simulink model "PHASE6_ASHUGANJ_CCPP_CLOSED_LOOP_TRIP"  (R2024a)
settings: Solver=FixedStepDiscrete  StartTime=0  StopTime=2  FixedStep=5e-05  RelTol=1e-3
PostLoadFcn:
  | p6startupdir=fileparts(get_param(bdroot,'FileName')); while ~isfile(fullfile(p6startupdir,'scripts','setup_phase6_workspace.m')), p6startupparent=fileparts(p6startupdir); assert(~strcmp(p6startupparent,p6startupdir),'Phase6:MissingScripts','Cannot locate the Phase6 scripts folder.'); p6startupdir=p6startupparent; end; addpath(fullfile(p6startupdir,'scripts')); setup_phase6_workspace; clear p6startupdir p6startupparent;
  | phase6_color_wires(bdroot);
StartFcn:
  | phase6_color_wires(bdroot);
StopFcn:
  | phase6_color_wires(bdroot);
model workspace (MAT data in the model file):
  C : object (value not decoded)
  D : object (value not decoded)
  P : object (value not decoded)
  Phase6BuildInfo : object (value not decoded)
  Phase6LoadFlow : object (value not decoded)
  Phase6Metadata : object (value not decoded)
  R : object (value not decoded)
  S : object (value not decoded)
symbols that are objects in the model workspace (value not decoded): C, D, R, S
undefined symbols (not defined in the file): D1, Delta
libraries: spsThreePhaseVIMeasurementLib x18, spsThreePhaseFaultLib x7, spsThreePhaseBreakerLib x5, spsThreePhaseParallelRLCLoadLib x4, spsThreePhasePISectionLineLib x4, spsThreePhaseTransformerTwoWindingsLib x3, spsGroundLib x3, spsSeriesRLCBranchLib x3, spsGroundingTransformerLib x1, spsCurrentMeasurementLib x1, spsSynchronousMachinepuStandardLib x1, spsThreePhaseMutualInductanceZ1Z0Lib x1
(part 2 of 2)

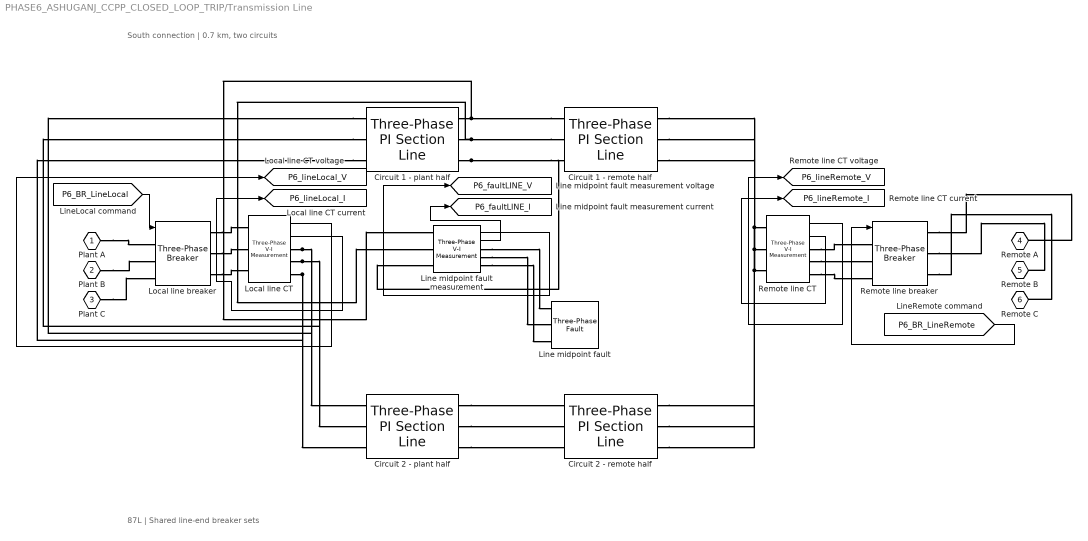
== system PHASE6_ASHUGANJ_CCPP_CLOSED_LOOP_TRIP/Transmission Line ==
  note: South connection | 0.7 km, two circuits
  note: 87L | Shared line-end breaker sets
  Circuit 1 - plant half : spsThreePhasePISectionLineLib/Three-Phase PI Section Line  LConnTagsString=a|b|c  RConnTagsString=A|B|C  Length=0.35  Frequency=50  Resistances=[0.08 0.25]  Inductances=[0.00111408460164327 0.00381971863420549]  Capacitances=[1.33690152197192e-08 8.91267681314614e-09]
  Circuit 1 - remote half : spsThreePhasePISectionLineLib/Three-Phase PI Section Line  LConnTagsString=a|b|c  RConnTagsString=A|B|C  Length=0.35  Frequency=50  Resistances=[0.08 0.25]  Inductances=[0.00111408460164327 0.00381971863420549]  Capacitances=[1.33690152197192e-08 8.91267681314614e-09]
  Circuit 2 - plant half : spsThreePhasePISectionLineLib/Three-Phase PI Section Line  LConnTagsString=a|b|c  RConnTagsString=A|B|C  Length=0.35  Frequency=50  Resistances=[0.08 0.25]  Inductances=[0.00111408460164327 0.00381971863420549]  Capacitances=[1.33690152197192e-08 8.91267681314614e-09]
  Circuit 2 - remote half : spsThreePhasePISectionLineLib/Three-Phase PI Section Line  LConnTagsString=a|b|c  RConnTagsString=A|B|C  Length=0.35  Frequency=50  Resistances=[0.08 0.25]  Inductances=[0.00111408460164327 0.00381971863420549]  Capacitances=[1.33690152197192e-08 8.91267681314614e-09]
  Line midpoint fault : spsThreePhaseFaultLib/Three-Phase Fault  InitialStates=0  FaultA=on  FaultB=on  FaultC=on  GroundFault=off  SwitchTimes=[1000000 1000001]  External=off  SwitchStatus=NaN  FaultResistance=0.01  GroundResistance=0.01  SnubberResistance=1000000000  SnubberCapacitance=inf  Measurements=None
  Line midpoint fault measurement : spsThreePhaseVIMeasurementLib/Three-Phase V-I Measurement  VoltageMeasurement=phase-to-ground  SetLabelV=off  LabelV=Vabc  Vpu=off  VpuLL=off  CurrentMeasurement=yes  SetLabelI=off  LabelI=Iabc  Ipu=off  Pbase=100e6  Vbase=500e3  OutputType=Complex  PhasorSimulation=off  PSBequivalent=0
  Local line CT : spsThreePhaseVIMeasurementLib/Three-Phase V-I Measurement  VoltageMeasurement=phase-to-ground  SetLabelV=off  LabelV=Vabc  Vpu=off  VpuLL=off  CurrentMeasurement=yes  SetLabelI=off  LabelI=Iabc  Ipu=off  Pbase=100e6  Vbase=500e3  OutputType=Complex  PhasorSimulation=off  PSBequivalent=0
  Local line breaker : spsThreePhaseBreakerLib/Three-Phase Breaker  InitialState=closed  SwitchA=on  SwitchB=on  SwitchC=on  SwitchTimes="[1/60  5/60]"  External=on  BreakerResistance=0.0001  SnubberResistance=1000000  SnubberCapacitance=inf  Measurements=None
  Remote line CT : spsThreePhaseVIMeasurementLib/Three-Phase V-I Measurement  VoltageMeasurement=phase-to-ground  SetLabelV=off  LabelV=Vabc  Vpu=off  VpuLL=off  CurrentMeasurement=yes  SetLabelI=off  LabelI=Iabc  Ipu=off  Pbase=100e6  Vbase=500e3  OutputType=Complex  PhasorSimulation=off  PSBequivalent=0
  Remote line breaker : spsThreePhaseBreakerLib/Three-Phase Breaker  InitialState=closed  SwitchA=on  SwitchB=on  SwitchC=on  SwitchTimes="[1/60  5/60]"  External=on  BreakerResistance=0.0001  SnubberResistance=1000000  SnubberCapacitance=inf  Measurements=None
  Plant A : PMIOPort  Side=Left
  Plant B : PMIOPort  Port=2  Side=Left
  Plant C : PMIOPort  Port=3  Side=Left
  Remote A : PMIOPort  Port=4  Side=Right
  Remote B : PMIOPort  Port=5  Side=Right
  Remote C : PMIOPort  Port=6  Side=Right
  tag scope: P6_faultLINE_I=global, P6_faultLINE_V=global, P6_lineLocal_I=global, P6_lineLocal_V=global, P6_lineRemote_I=global, P6_lineRemote_V=global
  wires:
  [P6_BR_LineLocal] -> Local line breaker/1
  Local line CT/1 -> [P6_lineLocal_V]
  Local line CT/2 -> [P6_lineLocal_I]
  Remote line CT/1 -> [P6_lineRemote_V]
  Remote line CT/2 -> [P6_lineRemote_I]
  [P6_BR_LineRemote] -> Remote line breaker/1
  Line midpoint fault measurement/1 -> [P6_faultLINE_V]
  Line midpoint fault measurement/2 -> [P6_faultLINE_I]
  connections:
  Plant A/RConn1 -- Local line breaker/LConn1
  Plant B/RConn1 -- Local line breaker/LConn2
  Plant C/RConn1 -- Local line breaker/LConn3
  Local line breaker/RConn1 -- Local line CT/LConn1
  Local line breaker/RConn2 -- Local line CT/LConn2
  Local line breaker/RConn3 -- Local line CT/LConn3
  Remote line CT/RConn1 -- Remote line breaker/LConn1
  Remote line CT/RConn2 -- Remote line breaker/LConn2
  Remote line CT/RConn3 -- Remote line breaker/LConn3
  Remote line breaker/RConn1 -- Remote A/RConn1
  Remote line breaker/RConn2 -- Remote B/RConn1
  Remote line breaker/RConn3 -- Remote C/RConn1
  Circuit 1 - plant half/LConn1 -- Local line CT/RConn1 -- Circuit 2 - plant half/LConn1
  Circuit 1 - plant half/LConn2 -- Local line CT/RConn2 -- Circuit 2 - plant half/LConn2
  Circuit 1 - plant half/LConn3 -- Local line CT/RConn3 -- Circuit 2 - plant half/LConn3
  Circuit 1 - remote half/LConn1 -- Circuit 1 - plant half/RConn1 -- Line midpoint fault measurement/LConn1
  Circuit 1 - remote half/LConn2 -- Circuit 1 - plant half/RConn2 -- Line midpoint fault measurement/LConn2
  Circuit 1 - remote half/LConn3 -- Circuit 1 - plant half/RConn3 -- Line midpoint fault measurement/LConn3
  Remote line CT/LConn1 -- Circuit 1 - remote half/RConn1 -- Circuit 2 - remote half/RConn1
  Remote line CT/LConn2 -- Circuit 1 - remote half/RConn2 -- Circuit 2 - remote half/RConn2
  Remote line CT/LConn3 -- Circuit 1 - remote half/RConn3 -- Circuit 2 - remote half/RConn3
  Line midpoint fault measurement/RConn1 -- Line midpoint fault/LConn1
  Line midpoint fault measurement/RConn2 -- Line midpoint fault/LConn2
  Line midpoint fault measurement/RConn3 -- Line midpoint fault/LConn3
  Circuit 2 - plant half/RConn1 -- Circuit 2 - remote half/LConn1
  Circuit 2 - plant half/RConn2 -- Circuit 2 - remote half/LConn2
  Circuit 2 - plant half/RConn3 -- Circuit 2 - remote half/LConn3

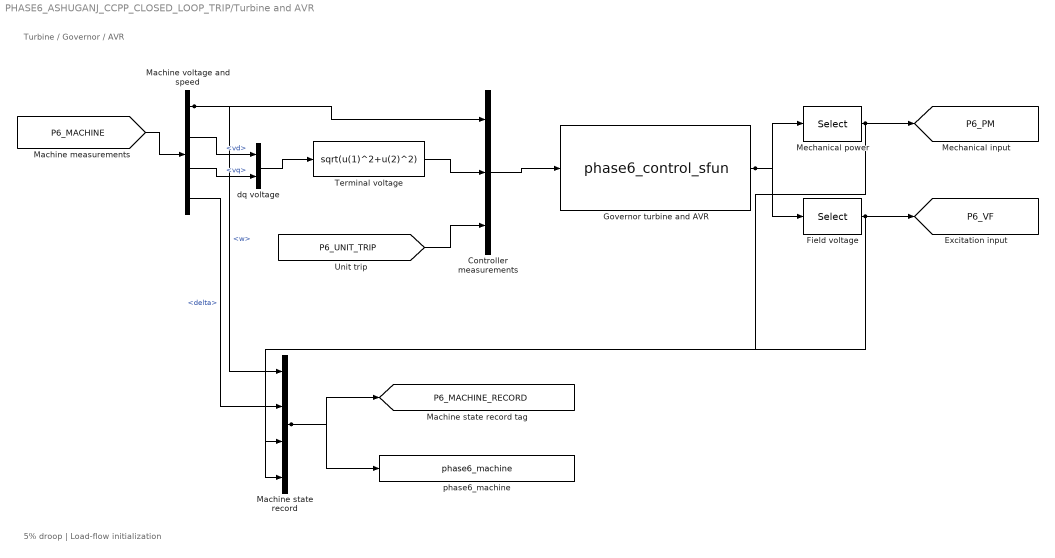
== system PHASE6_ASHUGANJ_CCPP_CLOSED_LOOP_TRIP/Turbine and AVR ==
  note: Turbine / Governor / AVR
  note: 5% droop | Load-flow initialization
  Controller measurements : Mux  Inputs=3
  Field voltage : Selector  IndexOptions=Index vector (dialog)  Indices=2  OutputSizes=1
  Governor turbine and AVR : M-S-Function  FunctionName=phase6_control_sfun  Parameters=C
  Machine state record : Mux
  Machine voltage and speed : BusSelector  OutputSignals=w,vd,vq,delta
  Mechanical power : Selector  IndexOptions=Index vector (dialog)  Indices=1  OutputSizes=1
  Terminal voltage : Fcn  Expr=sqrt(u(1)^2+u(2)^2)
  dq voltage : Mux  Inputs=2
  phase6_machine : ToWorkspace  VariableName=phase6_machine  SaveFormat=Timeseries  SampleTime=-1
  tag scope: P6_MACHINE_RECORD=global, P6_PM=global, P6_VF=global
  wires:
  [P6_MACHINE] -> Machine voltage and speed/1
  Machine voltage and speed/2 -> dq voltage/1  "<vd>"
  Machine voltage and speed/3 -> dq voltage/2  "<vq>"
  dq voltage/1 -> Terminal voltage/1
  Machine voltage and speed/1 -> Controller measurements/1, Machine state record/1  "<w>"
  Terminal voltage/1 -> Controller measurements/2
  [P6_UNIT_TRIP] -> Controller measurements/3
  Controller measurements/1 -> Governor turbine and AVR/1
  Governor turbine and AVR/1 -> Mechanical power/1, Field voltage/1
  Mechanical power/1 -> [P6_PM], Machine state record/3
  Field voltage/1 -> [P6_VF], Machine state record/4
  Machine voltage and speed/4 -> Machine state record/2  "<delta>"
  Machine state record/1 -> [P6_MACHINE_RECORD], phase6_machine/1

== system PHASE6_ASHUGANJ_CCPP_CLOSED_LOOP_TRIP/Auxiliaries/B6.6 Auxiliary 6.6 kV bus ==
  A1 : PMIOPort  Side=Left
  B1 : PMIOPort  Port=2  Side=Left
  C1 : PMIOPort  Port=3  Side=Left
  A2 : PMIOPort  Port=4  Side=Right
  B2 : PMIOPort  Port=5  Side=Right
  C2 : PMIOPort  Port=6  Side=Right
  connections:
  A1/RConn1 -- A2/RConn1
  B1/RConn1 -- B2/RConn1
  C1/RConn1 -- C2/RConn1

== system PHASE6_ASHUGANJ_CCPP_CLOSED_LOOP_TRIP/Grid/BGRID_230 PGCB 230 kV bus ==
  A1 : PMIOPort  Side=Left
  B1 : PMIOPort  Port=2  Side=Left
  C1 : PMIOPort  Port=3  Side=Left
  A2 : PMIOPort  Port=4  Side=Right
  B2 : PMIOPort  Port=5  Side=Right
  C2 : PMIOPort  Port=6  Side=Right
  connections:
  A1/RConn1 -- A2/RConn1
  B1/RConn1 -- B2/RConn1
  C1/RConn1 -- C2/RConn1

== system PHASE6_ASHUGANJ_CCPP_CLOSED_LOOP_TRIP/Measurements/Auxiliary and neutral ==
  Voltage and current channels : Mux  Inputs=6
  Measured abc : Outport
  wires:
  [P6_aux_V] -> Voltage and current channels/1
  [P6_aux_I] -> Voltage and current channels/2
  [P6_grid_V] -> Voltage and current channels/3
  [P6_grid_I] -> Voltage and current channels/4
  [P6_neutral_V] -> Voltage and current channels/5
  [P6_neutral_I] -> Voltage and current channels/6
  Voltage and current channels/1 -> Measured abc/1

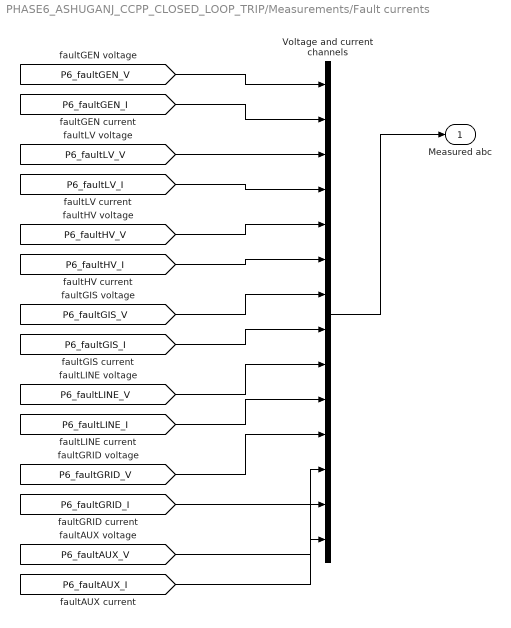
== system PHASE6_ASHUGANJ_CCPP_CLOSED_LOOP_TRIP/Measurements/Fault currents ==
  Voltage and current channels : Mux  Inputs=14
  Measured abc : Outport
  wires:
  [P6_faultGEN_V] -> Voltage and current channels/1
  [P6_faultGEN_I] -> Voltage and current channels/2
  [P6_faultLV_V] -> Voltage and current channels/3
  [P6_faultLV_I] -> Voltage and current channels/4
  [P6_faultHV_V] -> Voltage and current channels/5
  [P6_faultHV_I] -> Voltage and current channels/6
  [P6_faultGIS_V] -> Voltage and current channels/7
  [P6_faultGIS_I] -> Voltage and current channels/8
  [P6_faultLINE_V] -> Voltage and current channels/9
  [P6_faultLINE_I] -> Voltage and current channels/10
  [P6_faultGRID_V] -> Voltage and current channels/11
  [P6_faultGRID_I] -> Voltage and current channels/12
  [P6_faultAUX_V] -> Voltage and current channels/13
  [P6_faultAUX_I] -> Voltage and current channels/14
  Voltage and current channels/1 -> Measured abc/1

== system PHASE6_ASHUGANJ_CCPP_CLOSED_LOOP_TRIP/Measurements/Generator and transformer ==
  Voltage and current channels : Mux  Inputs=8
  Measured abc : Outport
  wires:
  [P6_genInner_V] -> Voltage and current channels/1
  [P6_genInner_I] -> Voltage and current channels/2
  [P6_genTerminal_V] -> Voltage and current channels/3
  [P6_genTerminal_I] -> Voltage and current channels/4
  [P6_gsutLV_V] -> Voltage and current channels/5
  [P6_gsutLV_I] -> Voltage and current channels/6
  [P6_gsutHV_V] -> Voltage and current channels/7
  [P6_gsutHV_I] -> Voltage and current channels/8
  Voltage and current channels/1 -> Measured abc/1

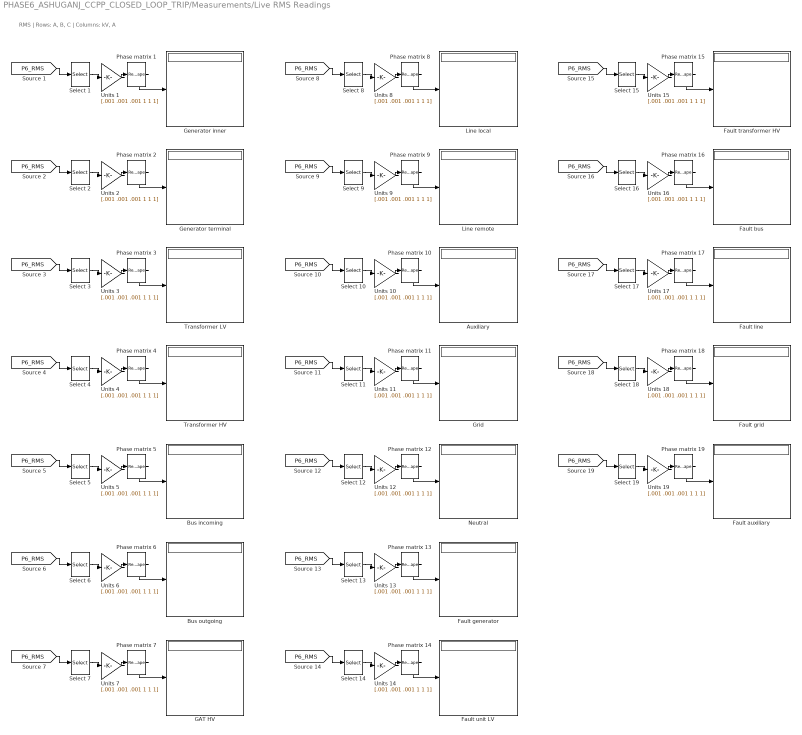
== system PHASE6_ASHUGANJ_CCPP_CLOSED_LOOP_TRIP/Measurements/Live RMS Readings ==
  note: RMS | Rows: A, B, C | Columns: kV, A
  Auxiliary : Display
  Bus incoming : Display
  Bus outgoing : Display
  Fault auxiliary : Display
  Fault bus : Display
  Fault generator : Display
  Fault grid : Display
  Fault line : Display
  Fault transformer HV : Display
  Fault unit LV : Display
  GAT HV : Display
  Generator inner : Display
  Generator terminal : Display
  Grid : Display
  Line local : Display
  Line remote : Display
  Neutral : Display
  Phase matrix {1..19} (19 alike) : Reshape  OutputDimensionality=Customize  OutputDimensions=[3 2]
  Select 1 : Selector  InputPortWidth=114  IndexOptions=Index vector (dialog)  Indices=[1 2 3 4 5 6]  OutputSizes=1
  Select 10 : Selector  InputPortWidth=114  IndexOptions=Index vector (dialog)  Indices=[55 56 57 58 59 60]  OutputSizes=1
  Select 11 : Selector  InputPortWidth=114  IndexOptions=Index vector (dialog)  Indices=[61 62 63 64 65 66]  OutputSizes=1
  Select 12 : Selector  InputPortWidth=114  IndexOptions=Index vector (dialog)  Indices=[67 68 69 70 71 72]  OutputSizes=1
  Select 13 : Selector  InputPortWidth=114  IndexOptions=Index vector (dialog)  Indices=[73 74 75 76 77 78]  OutputSizes=1
  Select 14 : Selector  InputPortWidth=114  IndexOptions=Index vector (dialog)  Indices=[79 80 81 82 83 84]  OutputSizes=1
  Select 15 : Selector  InputPortWidth=114  IndexOptions=Index vector (dialog)  Indices=[85 86 87 88 89 90]  OutputSizes=1
  Select 16 : Selector  InputPortWidth=114  IndexOptions=Index vector (dialog)  Indices=[91 92 93 94 95 96]  OutputSizes=1
  Select 17 : Selector  InputPortWidth=114  IndexOptions=Index vector (dialog)  Indices=[97 98 99 100 101 102]  OutputSizes=1
  Select 18 : Selector  InputPortWidth=114  IndexOptions=Index vector (dialog)  Indices=[103 104 105 106 107 108]  OutputSizes=1
  Select 19 : Selector  InputPortWidth=114  IndexOptions=Index vector (dialog)  Indices=[109 110 111 112 113 114]  OutputSizes=1
  Select 2 : Selector  InputPortWidth=114  IndexOptions=Index vector (dialog)  Indices=[7 8 9 10 11 12]  OutputSizes=1
  Select 3 : Selector  InputPortWidth=114  IndexOptions=Index vector (dialog)  Indices=[13 14 15 16 17 18]  OutputSizes=1
  Select 4 : Selector  InputPortWidth=114  IndexOptions=Index vector (dialog)  Indices=[19 20 21 22 23 24]  OutputSizes=1
  Select 5 : Selector  InputPortWidth=114  IndexOptions=Index vector (dialog)  Indices=[25 26 27 28 29 30]  OutputSizes=1
  Select 6 : Selector  InputPortWidth=114  IndexOptions=Index vector (dialog)  Indices=[31 32 33 34 35 36]  OutputSizes=1
  Select 7 : Selector  InputPortWidth=114  IndexOptions=Index vector (dialog)  Indices=[37 38 39 40 41 42]  OutputSizes=1
  Select 8 : Selector  InputPortWidth=114  IndexOptions=Index vector (dialog)  Indices=[43 44 45 46 47 48]  OutputSizes=1
  Select 9 : Selector  InputPortWidth=114  IndexOptions=Index vector (dialog)  Indices=[49 50 51 52 53 54]  OutputSizes=1
  Transformer HV : Display
  Transformer LV : Display
  Units {1..19} (19 alike) : Gain  Gain=[.001 .001 .001 1 1 1]
  wires:
  [P6_RMS] -> Select 1/1
  Select 1/1 -> Units 1/1
  [P6_RMS] -> Select 2/1
  Select 2/1 -> Units 2/1
  [P6_RMS] -> Select 3/1
  Select 3/1 -> Units 3/1
  [P6_RMS] -> Select 4/1
  Select 4/1 -> Units 4/1
  [P6_RMS] -> Select 5/1
  Select 5/1 -> Units 5/1
  [P6_RMS] -> Select 6/1
  Select 6/1 -> Units 6/1
  [P6_RMS] -> Select 7/1
  Select 7/1 -> Units 7/1
  [P6_RMS] -> Select 8/1
  Select 8/1 -> Units 8/1
  [P6_RMS] -> Select 9/1
  Select 9/1 -> Units 9/1
  [P6_RMS] -> Select 10/1
  Select 10/1 -> Units 10/1
  [P6_RMS] -> Select 11/1
  Select 11/1 -> Units 11/1
  [P6_RMS] -> Select 12/1
  Select 12/1 -> Units 12/1
  [P6_RMS] -> Select 13/1
  Select 13/1 -> Units 13/1
  [P6_RMS] -> Select 14/1
  Select 14/1 -> Units 14/1
  [P6_RMS] -> Select 15/1
  Select 15/1 -> Units 15/1
  [P6_RMS] -> Select 16/1
  Select 16/1 -> Units 16/1
  [P6_RMS] -> Select 17/1
  Select 17/1 -> Units 17/1
  [P6_RMS] -> Select 18/1
  Select 18/1 -> Units 18/1
  [P6_RMS] -> Select 19/1
  Select 19/1 -> Units 19/1
  Units 1/1 -> Phase matrix 1/1
  Phase matrix 1/1 -> Generator inner/1
  Units 2/1 -> Phase matrix 2/1
  Phase matrix 2/1 -> Generator terminal/1
  Units 3/1 -> Phase matrix 3/1
  Phase matrix 3/1 -> Transformer LV/1
  Units 4/1 -> Phase matrix 4/1
  Phase matrix 4/1 -> Transformer HV/1
  Units 5/1 -> Phase matrix 5/1
  Phase matrix 5/1 -> Bus incoming/1
  Units 6/1 -> Phase matrix 6/1
  Phase matrix 6/1 -> Bus outgoing/1
  Units 7/1 -> Phase matrix 7/1
  Phase matrix 7/1 -> GAT HV/1
  Units 8/1 -> Phase matrix 8/1
  Phase matrix 8/1 -> Line local/1
  Units 9/1 -> Phase matrix 9/1
  Phase matrix 9/1 -> Line remote/1
  Units 10/1 -> Phase matrix 10/1
  Phase matrix 10/1 -> Auxiliary/1
  Units 11/1 -> Phase matrix 11/1
  Phase matrix 11/1 -> Grid/1
  Units 12/1 -> Phase matrix 12/1
  Phase matrix 12/1 -> Neutral/1
  Units 13/1 -> Phase matrix 13/1
  Phase matrix 13/1 -> Fault generator/1
  Units 14/1 -> Phase matrix 14/1
  Phase matrix 14/1 -> Fault unit LV/1
  Units 15/1 -> Phase matrix 15/1
  Phase matrix 15/1 -> Fault transformer HV/1
  Units 16/1 -> Phase matrix 16/1
  Phase matrix 16/1 -> Fault bus/1
  Units 17/1 -> Phase matrix 17/1
  Phase matrix 17/1 -> Fault line/1
  Units 18/1 -> Phase matrix 18/1
  Phase matrix 18/1 -> Fault grid/1
  Units 19/1 -> Phase matrix 19/1
  Phase matrix 19/1 -> Fault auxiliary/1

== system PHASE6_ASHUGANJ_CCPP_CLOSED_LOOP_TRIP/Measurements/Switchyard and line ==
  Voltage and current channels : Mux  Inputs=10
  Measured abc : Outport
  wires:
  [P6_busIn_V] -> Voltage and current channels/1
  [P6_busIn_I] -> Voltage and current channels/2
  [P6_busOut_V] -> Voltage and current channels/3
  [P6_busOut_I] -> Voltage and current channels/4
  [P6_gatHV_V] -> Voltage and current channels/5
  [P6_gatHV_I] -> Voltage and current channels/6
  [P6_lineLocal_V] -> Voltage and current channels/7
  [P6_lineLocal_I] -> Voltage and current channels/8
  [P6_lineRemote_V] -> Voltage and current channels/9
  [P6_lineRemote_I] -> Voltage and current channels/10
  Voltage and current channels/1 -> Measured abc/1

== system PHASE6_ASHUGANJ_CCPP_CLOSED_LOOP_TRIP/Switchyard/B_230 GIS 230 kV bus ==
  A1 : PMIOPort  Side=Left
  B1 : PMIOPort  Port=2  Side=Left
  C1 : PMIOPort  Port=3  Side=Left
  A2 : PMIOPort  Port=4  Side=Right
  B2 : PMIOPort  Port=5  Side=Right
  C2 : PMIOPort  Port=6  Side=Right
  connections:
  A1/RConn1 -- A2/RConn1
  B1/RConn1 -- B2/RConn1
  C1/RConn1 -- C2/RConn1
